simulink model "BE6_7et8_obser_auto_simu"  (R2018b)
settings: Solver=VariableStepAuto  StartTime=0.0  StopTime=20  RelTol=1e-3
values from neighbouring files (symbols this model uses):
  A = [1  a1 a2]    [BE2_auto.m]    (also in BE6_7et8_auto.m = [a1 0 0; 0 0 1; a2 a3 0]; BE_synthese.m = [-alpha1 0; alpha1 -alpha2])
  B = [0 b1 b2]    [BE2_auto.m]    (also in BE6_7et8_auto.m = [b1; 0; 0]; BE_synthese.m = [sigma0; 0])
  C = [0 1 0]    [BE6_7et8_auto.m]    (also in BE_synthese.m = [0 1])
  F = [Fe(1) Fe(2) Fe(3)]    [BE6_7et8_auto.m]    (also in BE_synthese.m = [Fe(1) Fe(2)])
  G = [Fe(4)]    [BE6_7et8_auto.m]    (also in BE_synthese.m = [Fe(3)])
  L = place(A',C',rts)'    [BE6_7et8_auto.m]    (also in BE_synthese.m = place(A',C',poles_cont)')
settings Model: Creator=piffercg  LastModifiedBy=piffercg

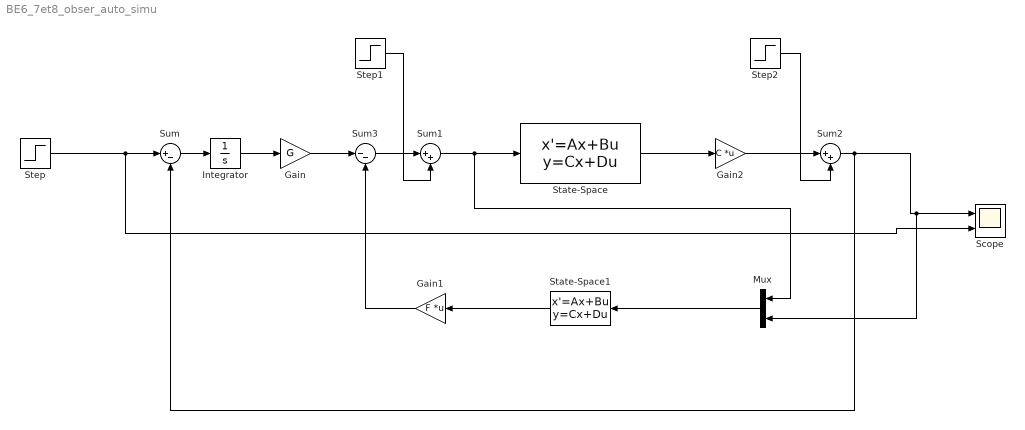
== system BE6_7et8_obser_auto_simu ==
  Gain : Gain  Gain=G
  Gain1 : Gain  Gain=F  Multiplication=Matrix(K*u)
  Gain2 : Gain  Gain=C  Multiplication=Matrix(K*u)
  Integrator : Integrator
  Mux : Mux  Inputs=2
  Scope : Scope  NumInputPorts=2
  State-Space : StateSpace  A=A  B=B  C=eye(2)  D=zeros(2,1)  InitialCondition=0
  State-Space1 : StateSpace  A=A-L*C  B=[B L]  C=eye(2)  D=zeros(2,2)  InitialCondition=0
  Step : Step  After=9  SampleTime=0
  Step1 : Step  Time=5  After=0  SampleTime=0
  Step2 : Step  Time=10  After=100  SampleTime=0
  Sum : Sum  Inputs=|+-
  Sum1 : Sum  Inputs=|++
  Sum2 : Sum  Inputs=|++
  Sum3 : Sum  Inputs=|--
  wires:
  Step/1 -> Sum/1, Scope/2
  Gain2/1 -> Sum2/1
  Step2/1 -> Sum2/2
  Step1/1 -> Sum1/2
  Gain1/1 -> Sum3/2
  Sum2/1 -> Scope/1, Mux/2, Sum/2
  State-Space/1 -> Gain2/1
  Sum1/1 -> Mux/1, State-Space/1
  State-Space1/1 -> Gain1/1
  Mux/1 -> State-Space1/1
  Integrator/1 -> Gain/1
  Sum/1 -> Integrator/1
  Gain/1 -> Sum3/1
  Sum3/1 -> Sum1/1
